simulink model "item4"  (R2013a)
settings: Solver=ode45  StartTime=0.0  StopTime=1.5  RelTol=1e-3
undefined symbols (not defined in the file): alpha, alpha2
libraries: powerlib x13
settings Model: Creator=Guilherme  LastModifiedBy=Guilherme

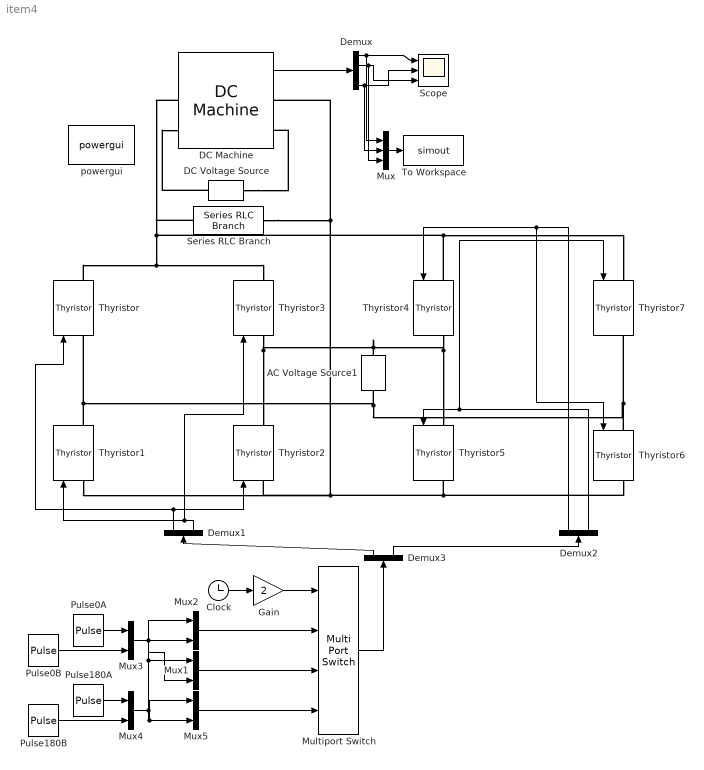
== system item4 ==
  AC Voltage Source1 : powerlib/Electrical Sources/AC Voltage Source  Amplitude=24*sqrt(2)  Phase=0  Frequency=60  SampleTime=0  Measurements=Voltage
  Clock : Clock
  DC Machine : powerlib/Machines/DC Machine  PresetModel=No  MechanicalLoad=Torque TL  FieldType=Wound  ShowDetailedParameters=on  RLa="[ 1.6  6.67e-4 ]"  RLf=[ 1 0 ]  Laf=0.038  MachineConstant=Torque constant (N.m/A)  Ke=1.8  Kt=1.8  J=1.1e-4  Bm=1.24e-4  Tf=0  w0=1  Ifinit=1  TsPowergui=0  TsBlock=-1
  DC Voltage Source : powerlib/Electrical Sources/DC Voltage Source  Amplitude=1  Measurements=None
  Demux : Demux
  Demux1 : Demux  Outputs=2
  Demux2 : Demux  Outputs=2
  Demux3 : Demux  Outputs=2
  Gain : Gain  Gain=2
  Multiport Switch : MultiPortSwitch  DataPortOrder=Zero-based contiguous  DiagnosticForDefault=None
  Mux : Mux  Inputs=3
  Mux{1..5} (5 alike) : Mux  Inputs=2
  Pulse0A : DiscretePulseGenerator  PulseType=Time based  Amplitude=3  Period=1/60  PulseWidth=10  PhaseDelay=1/60*(alpha/360)
  Pulse0B : DiscretePulseGenerator  PulseType=Time based  Amplitude=3  Period=1/60  PulseWidth=10  PhaseDelay=1/60*((alpha+180)/360)
  Pulse180A : DiscretePulseGenerator  PulseType=Time based  Amplitude=3  Period=1/60  PulseWidth=10  PhaseDelay=1/60*(alpha2/360)
  Pulse180B : DiscretePulseGenerator  PulseType=Time based  Amplitude=3  Period=1/60  PulseWidth=10  PhaseDelay=1/60*((alpha2+180)/360)
  Scope : Scope  NumInputPorts=3
      settings: YMin=0~-0.05~-2.5  YMax=70~0.75~20
  Series RLC Branch : powerlib/Elements/Series RLC Branch  LConnTagsString=__new0  RConnTagsString=__new0  BranchType=C  Resistance=1  Inductance=1e-3  SetiL0=off  InitialCurrent=0  Capacitance=1  Setx0=off  InitialVoltage=0  Measurements=None
  Thyristor{,1..7} (8 alike) : powerlib/Power Electronics/Thyristor  Ron=0.001  Lon=0  Vf=0.8  IC=0  Rs=500  Cs=250e-9  Measurements=on
  To Workspace : ToWorkspace  VariableName=simout  SampleTime=-1  SaveFormat=Timeseries
  powergui : powerlib/powergui  Priority=1  SimulationMode=Discrete  SolverType=Tustin  SampleTime=5e-6  frequency=60  SPID=off  DisableSnubberDevices=off  DisableRonSwitches=off  DisableVfSwitches=off  SwTol=0  Interpol=off  DisplayEquations=off  frequencyindice=0  Pbase=100e6  ErrMax=1e-4  Iterations=50  UnitsV=kV  UnitsW=MW  FunctionMessages=off  echomessages=off  HookPort=off  EnableUseOfTLC=off  x0status=blocks  RestoreLinks=warning  ResistiveCurrentMeasurement=off  Frange=[0:2:500]  Ylog=off  Xlog=on  ShowGrid=off  save=off  variable=ZData  ZoomFFT=off  StartTime=0.0  cycles=1  DisplayStyle=1  fundamental=60  FreqAxis=off  MaxFrequency=1000  frequencyindicesteady=1  RmsSteady=1  display=off  Ts=0  methode=off
  wires:
  DC Machine/1 -> Demux/1
  Demux/1 -> Scope/1, Mux/1
  Demux/4 -> Mux/2, Scope/2
  Demux/2 -> Mux/3, Scope/3
  Mux/1 -> To Workspace/1
  Demux1/1 -> Thyristor2/1, Thyristor/1
  Demux1/2 -> Thyristor1/1, Thyristor3/1
  Demux2/1 -> Thyristor4/1, Thyristor6/1
  Demux2/2 -> Thyristor5/1, Thyristor7/1
  Multiport Switch/1 -> Demux3/1
  Pulse0A/1 -> Mux3/1
  Pulse0B/1 -> Mux3/2
  Pulse180A/1 -> Mux4/1
  Pulse180B/1 -> Mux4/2
  Mux3/1 -> Mux1/2, Mux2/1
  Mux4/1 -> Mux5/2, Mux5/1, Mux1/1, Mux2/2
  Demux3/2 -> Demux2/1
  Demux3/1 -> Demux1/1
  Clock/1 -> Gain/1
  Gain/1 -> Multiport Switch/1
  Mux2/1 -> Multiport Switch/2
  Mux1/1 -> Multiport Switch/3
  Mux5/1 -> Multiport Switch/4
  connections:
  DC Voltage Source/RConn1 -- DC Machine/LConn2
  DC Voltage Source/LConn1 -- DC Machine/RConn2
  Thyristor4/LConn1 -- Thyristor7/LConn1 -- Thyristor/RConn1 -- Thyristor3/RConn1 -- DC Machine/LConn1 -- Series RLC Branch/LConn1
  Thyristor6/RConn1 -- Thyristor1/LConn1 -- Thyristor2/LConn1 -- Series RLC Branch/RConn1 -- DC Machine/RConn1 -- Thyristor5/RConn1
  Thyristor3/LConn1 -- Thyristor2/RConn1 -- Thyristor4/RConn1 -- Thyristor5/LConn1 -- AC Voltage Source1/LConn1
  Thyristor1/RConn1 -- Thyristor/LConn1 -- Thyristor7/RConn1 -- Thyristor6/LConn1 -- AC Voltage Source1/RConn1
